simulink model "trackBase1"  (R2019b)
settings: Solver=VariableStepAuto  StartTime=0.0  StopTime=100.0  RelTol=1e-3
settings Model: Creator=mansn  LastModifiedBy=mansn
settings SolverCC: AlgebraicLoopSolver=LineSearch

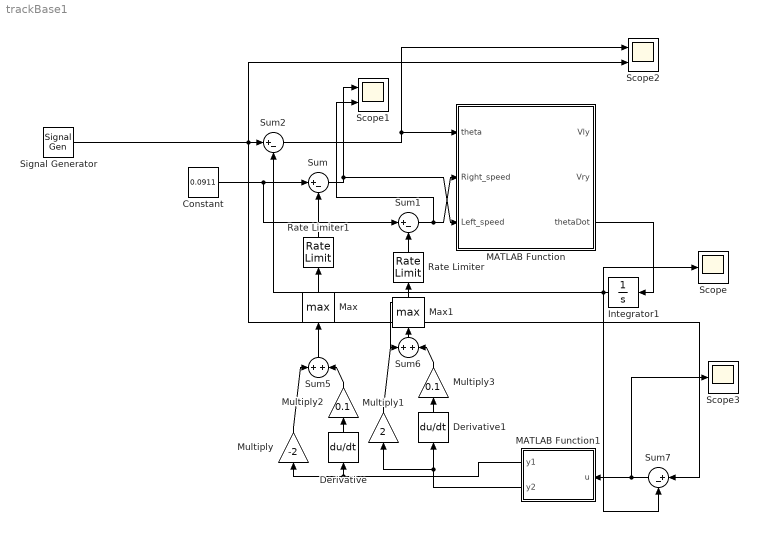
== system trackBase1 ==
  Constant : Constant  Value=0.0911
  Derivative : Derivative
  Derivative1 : Derivative
  Integrator1 : Integrator
  MATLAB Function : MATLAB Function  TreatAsAtomicUnit=on
  MATLAB Function1 : MATLAB Function  TreatAsAtomicUnit=on
  Max : MinMax  Function=max  OutMin=0  OutMax=0.0911*2
  Max1 : MinMax  Function=max  OutMin=0  OutMax=0.0911*2
  Multiply : Gain  Gain=-2
  Multiply1 : Gain  Gain=2
  Multiply2 : Gain  Gain=0.1
  Multiply3 : Gain  Gain=0.1
  Rate Limiter : RateLimiter  SampleTimeMode=inherited
  Rate Limiter1 : RateLimiter  SampleTimeMode=inherited
  Scope : Scope
  Scope1 : Scope  NumInputPorts=2
  Scope2 : Scope  NumInputPorts=2
  Scope3 : Scope
  Signal Generator : SignalGenerator  Frequency=0.1  Units=rad/sec
  Sum{,1..2,7} (4 alike) : Sum  Inputs=|+-
  Sum5 : Sum
  Sum6 : Sum
  wires:
  Sum/1 -> Scope1/1, MATLAB Function/3(Left_speed)
  Sum1/1 -> Scope1/2, MATLAB Function/2(Right_speed)
  Constant/1 -> Sum/1, Sum1/1
  Sum2/1 -> Scope2/1, MATLAB Function/1(theta)
  Integrator1/1 -> Scope/1, Sum2/2, Sum7/2
  Multiply/1 -> Sum5/1
  MATLAB Function1/1(y1) -> Multiply/1, Derivative/1
  Derivative/1 -> Multiply2/1
  Multiply2/1 -> Sum5/2
  Multiply1/1 -> Sum6/1
  Multiply3/1 -> Sum6/2
  Derivative1/1 -> Multiply3/1
  Sum6/1 -> Max1/1
  MATLAB Function1/2(y2) -> Multiply1/1, Derivative1/1
  Signal Generator/1 -> Sum7/1, Sum2/1, Scope2/2
  Sum7/1 -> Scope3/1, MATLAB Function1/1(u)
  MATLAB Function/3(thetaDot) -> Integrator1/1
  Sum5/1 -> Max/1
  Rate Limiter/1 -> Sum1/2
  Max1/1 -> Rate Limiter/1
  Max/1 -> Rate Limiter1/1
  Rate Limiter1/1 -> Sum/2

== matlab function trackBase1/MATLAB Function1 ==
  data: u input; y1 output; y2 output
function [y1, y2] = fcn(u)

if u<0
   y1=u;
   y2=0;
else
    y2=u;
    y1=0;
end

== matlab function trackBase1/MATLAB Function ==
  data: theta input; Right_speed input; Left_speed input; Vly output; Vry output; thetaDot output
function [Vly,Vry,thetaDot] = trackBase1(theta,Right_speed,Left_speed)

h=0.30;         % Length that the robot measures the angle at
L=0.1;          % Length from center of robot to the

%x0=sin(theta)*h;

% Speed for the motors in x - direction
Vlx=-Left_speed*cos(theta);
Vrx=-Right_speed*cos(theta);

% Speed for the motors in y - direction
Vly=Left_speed*sin(theta);
Vry=Right_speed*sin(theta);

% Total speed of the motor
%Vl=sqrt(abs(Vlx)^2+abs(Vly)^2);
%Vr=sqrt(abs(Vrx)^2+abs(Vry)^2);


thetaDot=(Vrx+Vry-Vlx-Vly)/(2*L);
